simulink model "TSCLAB_Modelv_12_PV"  (R2017a)
settings: Solver=VariableStepAuto  StartTime=0.0  StopTime=200  RelTol=1e-3
undefined symbols (not defined in the file): serial
libraries: instrumentlib x3
settings Model: Creator=vasanza  LastModifiedBy=vasan
settings DataIOCC: ReturnWorkspaceOutputs=on
settings SFSimCC: SimUseLocalCustomCode=on
settings RTWCC: RTWUseLocalCustomCode=on

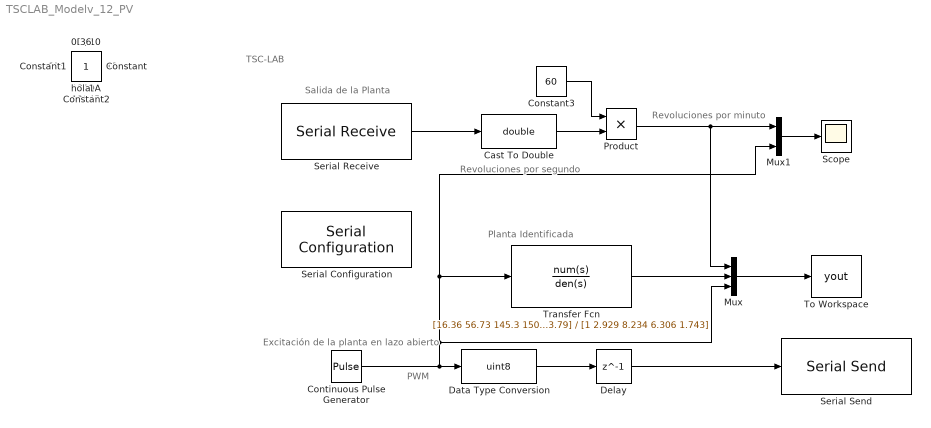
== system TSCLAB_Modelv_12_PV ==
  note: PWM
  note: Excitación de la planta en lazo abierto
  note: Planta Identificada
  note: Revoluciones por minuto
  note: Revoluciones por segundo
  note: Salida de la Planta
  note: TSC-LAB
  Cast To Double : DataTypeConversion  OutDataTypeStr=double
  Constant3 : Constant  Value=60
  Continuous Pulse Generator : DiscretePulseGenerator  PulseType=Time based  Amplitude=255  Period=24  PulseWidth=50
  Data Type Conversion : DataTypeConversion  OutDataTypeStr=uint8
  Delay : Delay  DelayLength=1  InitialCondition=0
  Mux : Mux  Inputs=3
  Mux1 : Mux  Inputs=2
  Product : Product
  Scope : Scope
  Serial Configuration : instrumentlib/Serial Configuration  Priority=-200000  ObjConstructor=serial('COM11');  ComPortMenu=COM11  ComPort=COM11  BaudRate=115200  DataBits=8  Parity=none  StopBits=1  ByteOrder=LittleEndian  FlowControl=none  Timeout=10
  Serial Receive : instrumentlib/Serial Receive  ObjConstructor=serial('COM11');  ComPortMenu=COM11  ComPort=COM11  DataType=uint8  Terminator=<none>  DataSize=[1 1]  EnableBlockingMode=on  ActionDataUnavailable=Output last received value  CustomValue=0  SampleTime=0.999
  Serial Send : instrumentlib/Serial Send  ObjConstructor=serial('COM11');  ComPortMenu=COM11  ComPort=COM11  Terminator=<none>  EnableBlockingMode=on
  To Workspace : ToWorkspace  VariableName=yout  SampleTime=-1
      settings: Save2DSignal=2-D array (concatenate along first dimension)
  Transfer Fcn : TransferFcn  Numerator=[16.36 56.73 145.3 150 53.79]  Denominator=[1 2.929 8.234 6.306 1.743]
  $ : Constant  IOType=siggen  Value=36
  , : Constant  IOType=siggen  Value=44
  {0,10,255,311,12345} (5 alike) : Constant  IOType=siggen
  0A : Constant  IOType=siggen  Value=10
  0D : Constant  IOType=siggen  Value=13
  13 : Constant  IOType=siggen  Value=13
  36 : Constant  IOType=siggen  Value=36
  Constant : Constant  IOType=siggen
  Constant1 : Constant  IOType=siggen
  Constant2 : Constant  IOType=siggen
  hola : Constant  IOType=siggen
  wires:
  Mux/1 -> To Workspace/1
  Transfer Fcn/1 -> Mux/2
  Data Type Conversion/1 -> Delay/1
  Delay/1 -> Serial Send/1
  Serial Receive/1 -> Cast To Double/1
  Mux1/1 -> Scope/1
  Continuous Pulse Generator/1 -> Data Type Conversion/1, Mux/3, Transfer Fcn/1, Mux1/2
  Cast To Double/1 -> Product/2
  Constant3/1 -> Product/1
  Product/1 -> Mux/1, Mux1/1
